simulink model "ActuatorCommandRef"  (R2023b)
settings: Solver=FixedStepDiscrete  StartTime=0.0  StopTime=2  FixedStep=Sample_time  RelTol=1e-3
undefined symbols (not defined in the file): actuator_limit_deg, Sample_time
Description:
  | Referenced actuator-command magnitude saturation training component.
settings Model: DataDictionary=FCS_Data.sldd  Creator=Tyler  LastModifiedBy=Tyler
settings CodeAppCC: MaxIdLength=63

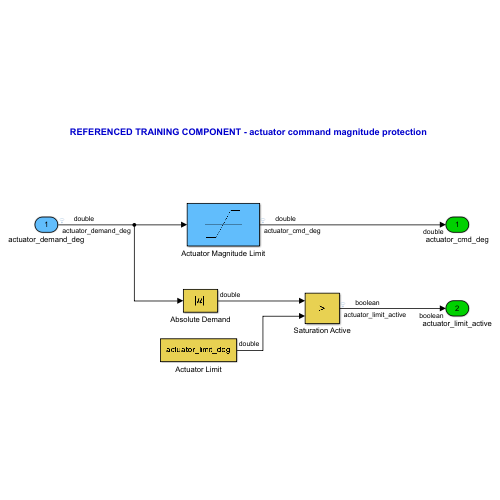
[thumbnail: Simulink's stored preview of the top-level diagram]
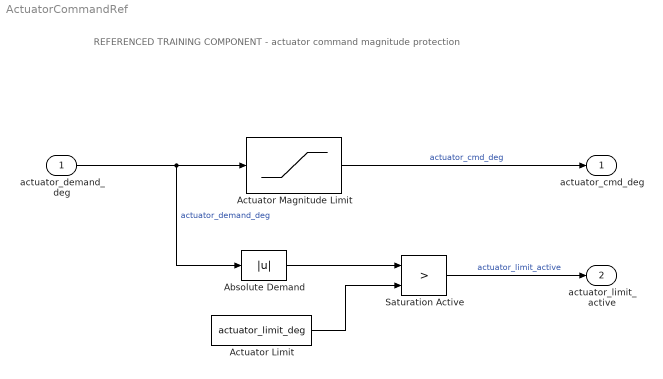
== system ActuatorCommandRef ==
  note: REFERENCED TRAINING COMPONENT - actuator command magnitude protection
  actuator_demand_deg : Inport  OutDataTypeStr=double  Unit=deg  SampleTime=Sample_time
  Absolute Demand : Abs  SaturateOnIntegerOverflow=off
  Actuator Limit : Constant  Value=actuator_limit_deg  OutDataTypeStr=double  SampleTime=Sample_time
  Actuator Magnitude Limit : Saturate  UpperLimit=actuator_limit_deg  LowerLimit=-actuator_limit_deg
  Saturation Active : RelationalOperator  Operator=>  OutDataTypeStr=boolean  RndMeth=Simplest  InputSameDT=off
  actuator_cmd_deg : Outport  OutDataTypeStr=double  Unit=deg
  actuator_limit_active : Outport  Port=2  OutDataTypeStr=boolean  Unit=1
  wires:
  actuator_demand_deg/1 -> Actuator Magnitude Limit/1, Absolute Demand/1  "actuator_demand_deg"
  Actuator Magnitude Limit/1 -> actuator_cmd_deg/1  "actuator_cmd_deg"
  Absolute Demand/1 -> Saturation Active/1
  Actuator Limit/1 -> Saturation Active/2
  Saturation Active/1 -> actuator_limit_active/1  "actuator_limit_active"
